simulink model "clamped_plate_KIRCHHOFF_superelem_aug"  (R2025b)
settings: Solver=VariableStepAuto  StartTime=0.0  StopTime=10  RelTol=1e-3
libraries: RCTblocks x1
settings Model: Creator=f.sanfedino  LastModifiedBy=andre
settings SolverCC: AlgebraicLoopSolver=TrustRegion
settings DataIOCC: ReturnWorkspaceOutputs=off
settings DebuggingCC: UnconnectedInputMsg=warning  UnconnectedOutputMsg=warning  UnconnectedLineMsg=warning
settings ModelReferenceCC: EnableRefExpFcnMdlSchedulingChecks=on
settings RTWCC: GPUComputeCapability=3.5  DLArmComputeVersion=19.05

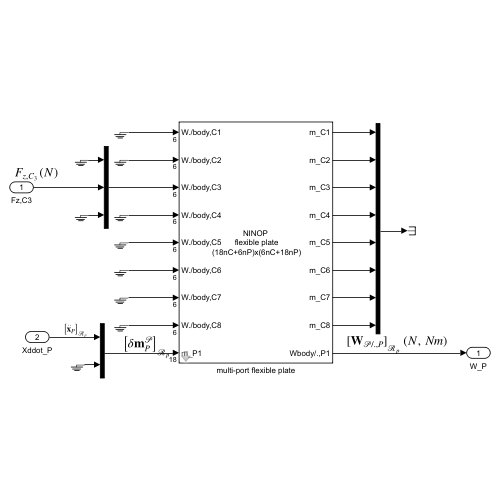
[thumbnail: Simulink's stored preview of the top-level diagram]
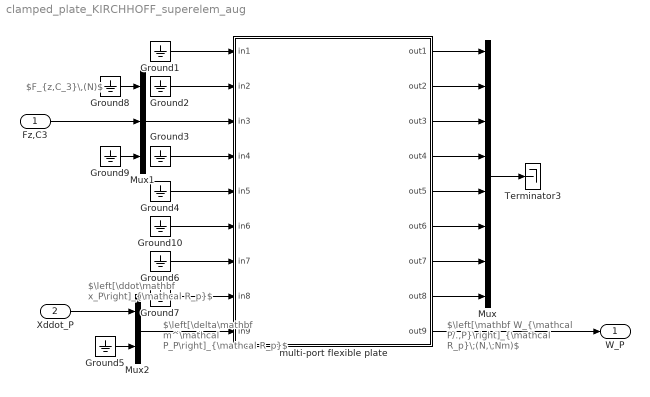
== system clamped_plate_KIRCHHOFF_superelem_aug ==
  note: $\left[\ddot\mathbf x_P\right]_{\mathcal R_p}$
  note: $F_{z,C_3}\,(N)$
  note: $\left[\mathbf W_{\mathcal P/.,P}\right]_{\mathcal R_p}\;(N,\;Nm)$
  note: $\left[\delta\mathbf m^\mathcal P_P\right]_{\mathcal R_p}$
  Fz,C3 : Inport
  Xddot_P : Inport  Port=2
  Ground{1..10} (10 alike) : Ground
  Mux : Mux  Inputs=18*ones(1,8)
  Mux1 : Mux  Inputs=[2 1 3]
  Mux2 : Mux  Inputs=[6 12]
  Terminator3 : Terminator
  multi-port flexible plate : Subsystem  mask(Multi-port flexible plate (18nC+6nP)x(6nC+18nP)){lx=1, ly=1, t=0.003, rho=2015.8, E=69.87e9, ni=0.5764, xi=0.001, i_nP=1, i_nC=8, OP1=[0;0.5;0], OP2=[1;1;0], OP3=[1;0;0], OP4=[1;1;0], OC1=[0;0;0], OC2=[0.5;0;0], OC3=[1;0;0], OC4=[0.5;0.5;0], OC5=[1;0.5;0], OC6=[0;1;0], OC7=[0.5;1;0], OC8=[1;1;0], RedSlowOn=off, uw_var=0, Nflex=0}
      mask prompts: lx "lenght along x (m)"; ly "length along y (m)"; t "thickness (m)"; rho "Mass density (Kg/m^3)"; E "Young modulus (N/m^2)"; ni "Poisson coefficient"; xi "damping coefficient"; i_nP "Number of parent (P) nodes (<5)"; i_nC "Number of child (C) nodes"; OP1 "OP1 (3x1 vector: [x;y;0], m)"; OP2 "OP2 (3x1 vectorr: [x;y;0], m)"; OP3 "OP3 (3x1 vectorr: [x;y;0], m)"; OP4 "OP4 (3x1 vectorr: [x;y;0], m)"; OC1 "OC1 (3x1 vectorr: [x;y;0], m)"; OC2 "OC2 (3x1 vectorr: [x;y;0], m)"; OC3 "OC3 (3x1 vectorr: [x;y;0], m)"; OC4 "OC4 (3x1 vectorr: [x;y;0], m)"; OC5 "OC5 (3x1 vectorr: [x;y;0], m)"; OC6 "OC6 (3x1 vectorr: [x;y;0], m)"; OC7 "OC7 (3x1 vector: [x;y;0],m)"; OC8 "OC8 (3x1 vector [x;y;0], m)"; RedSlowOn "Reduction of the 6*(nP-1) poles at 0 (due to loop closure constraints when nP>1)."; uw_var "uncertainty (%)"; Nflex "number of flexible modes (Nf, integer)"
      mask help:
      | (18nC+6nP)x(6nC+18nP) multi-port model of a uniform plate (in the x-y plane) between
      |   *  wrenches applied to the plate at the given nC child nodes (input) and motion vectors at these child nodes (output)
      |   *  motion vectors at the nP parent nodes (input)  and wrenches applied by this plate at these parent nodes (output)
      |  dynamic model of a uniform flexible plate (in the x-y plane),
      | in the plate reference frame (0,x,y,z)
      |
      | The plate is defined by:
      | * 0<x<lx
      | * 0<y<ly
      | * -t/2<z<t/2
      |
      | All parameters are expressed in the plate reference frame.
      | Dynamics in translations along x and y and rotation around z are assumed rigid.
      mask init:
      | MultiPortFlexiblePlateAug
      mask Help: web('DocPlate_joly.html','-browser')
      mask TypeOptions i_nP: 0 | 1 | 2 | 3 | 4
      mask TypeOptions i_nC: 0 | 1 | 2 | 3 | 4 | 5 | 6 | 7 | 8
      mask DialogControl ParameterGroupVar Prompt: Main parameters
      mask DialogControl Pport1 Prompt: P node #1
      mask DialogControl Pport2 Prompt: #2
      mask DialogControl Pport3 Prompt: #3
      mask DialogControl Pport4 Prompt: #4
      mask DialogControl Cport1 Prompt: C node #1
      mask DialogControl Cport2 Prompt: #2
      mask DialogControl Cport3 Prompt: #3
      mask DialogControl Cport4 Prompt: #4
      mask DialogControl Cport5 Prompt: #5
      mask DialogControl Cport6 Prompt: #6
      mask DialogControl Cport7 Prompt: #7
      mask DialogControl Cport8 Prompt: #8
      mask DialogControl Reduction Prompt: Optional Reduction
      mask DialogControl Container19 Prompt: Parametric uncertainties
      mask DialogControl Control8 Prompt: The uncertain parameters are the first Nf cantilevered frequencies of the plate when it is clamped at the first parent node (P1) or the last child node when the number of parent nodes is null.
      mask DialogControl Control4 Prompt: The uncertain frequency is named: 'w_name_i' where:
      mask DialogControl Control5 Prompt: * 'name' is the current block name (reduced to its alphanumeric characters).
      mask DialogControl Control6 Prompt: * 'i' is the flexible mode number (increasing frequency order)
      mask Display:
      | disp('NINOP\n flexible plate\n (18nC+6nP)x(6nC+18nP)')
      | if nC~=0
      |     for ii=1:nC
      |         port_label('input', ii, ['W./body,C',num2str(ii)])
      |         port_label('output',ii,['m_C',num2str(ii)])
      |     end
      | end
      | if nP~=0
      |     for ii=1:nP
      |         port_label('input', nC+ii, ['m_P',num2str(ii)])
      |         port_label('output',nC+ii,['Wbody/.,P',num2str(ii)])
      |     end
      | end
  W_P : Outport
  wires:
  Ground1/1 -> multi-port flexible plate/1(in1)
  Ground2/1 -> multi-port flexible plate/2(in2)
  Ground4/1 -> multi-port flexible plate/5(in5)
  Ground3/1 -> multi-port flexible plate/4(in4)
  Ground6/1 -> multi-port flexible plate/7(in7)
  Ground7/1 -> multi-port flexible plate/8(in8)
  multi-port flexible plate/1(out1) -> Mux/1
  multi-port flexible plate/2(out2) -> Mux/2
  multi-port flexible plate/3(out3) -> Mux/3
  multi-port flexible plate/4(out4) -> Mux/4
  multi-port flexible plate/5(out5) -> Mux/5
  multi-port flexible plate/6(out6) -> Mux/6
  multi-port flexible plate/7(out7) -> Mux/7
  multi-port flexible plate/8(out8) -> Mux/8
  multi-port flexible plate/9(out9) -> W_P/1
  Mux1/1 -> multi-port flexible plate/3(in3)
  Ground8/1 -> Mux1/1
  Ground9/1 -> Mux1/3
  Ground10/1 -> multi-port flexible plate/6(in6)
  Fz,C3/1 -> Mux1/2
  Mux/1 -> Terminator3/1
  Xddot_P/1 -> Mux2/1
  Ground5/1 -> Mux2/2
  Mux2/1 -> multi-port flexible plate/9(in9)

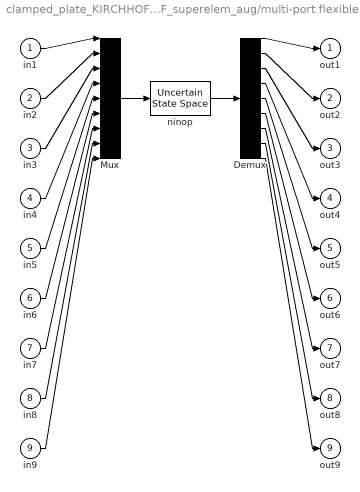
== system clamped_plate_KIRCHHOFF_superelem_aug/multi-port flexible plate ==
  in1 : Inport  PortDimensions=6
  in2 : Inport  Port=2  PortDimensions=6
  in3 : Inport  Port=3  PortDimensions=6
  in4 : Inport  Port=4  PortDimensions=6
  in5 : Inport  Port=5  PortDimensions=6
  in6 : Inport  Port=6  PortDimensions=6
  in7 : Inport  Port=7  PortDimensions=6
  in8 : Inport  Port=8  PortDimensions=6
  in9 : Inport  Port=9  PortDimensions=18
  Demux : Demux  Outputs=[18 18 18 18 18 18 18 18 6 ]
  Mux : Mux  Inputs=[6 6 6 6 6 6 6 6 18 ]
  ninop : RCTblocks/Uncertain State Space  Tag=USS  USystem=NINOP  UValue=[]  X0=[]  uX0=[]
  out1 : Outport
  out2 : Outport  Port=2
  out3 : Outport  Port=3
  out4 : Outport  Port=4
  out5 : Outport  Port=5
  out6 : Outport  Port=6
  out7 : Outport  Port=7
  out8 : Outport  Port=8
  out9 : Outport  Port=9
  wires:
  Mux/1 -> ninop/1
  ninop/1 -> Demux/1
  in1/1 -> Mux/1
  Demux/1 -> out1/1
  in2/1 -> Mux/2
  Demux/2 -> out2/1
  in3/1 -> Mux/3
  Demux/3 -> out3/1
  in4/1 -> Mux/4
  Demux/4 -> out4/1
  in5/1 -> Mux/5
  Demux/5 -> out5/1
  in6/1 -> Mux/6
  Demux/6 -> out6/1
  in7/1 -> Mux/7
  Demux/7 -> out7/1
  in8/1 -> Mux/8
  Demux/8 -> out8/1
  in9/1 -> Mux/9
  Demux/9 -> out9/1
